simulink model ""  (R2020b)
settings: Solver=VariableStepAuto  StartTime=0.0  StopTime=10  FixedStep=0.00001  MaxStep=1e-3  RelTol=1e-3
undefined symbols (not defined in the file): h
settings Model: Creator=jofr  LastModifiedBy=jofr
settings DataIOCC: LimitDataPoints=on  SaveFormat=Array  SignalLoggingSaveFormat=ModelDataLogs  ReturnWorkspaceOutputs=off
settings OptimizationCC: BlockReduction=off  BooleanDataType=off  LifeSpan=inf
settings DebuggingCC: SaveWithParameterizedLinksMsg=none  UnderspecifiedInitializationDetection=Classic  MergeDetectMultiDrivingBlocksExec=none  SignalResolutionControl=TryResolveAllWithWarning  MultiTaskDSMMsg=warning  MultiTaskCondExecSysMsg=none  SFUnexpectedBacktrackingDiag=warning  SFNoUnconditionalDefaultTransitionDiag=warning  SFExecutionAtInitializationDiag=none  ArithmeticOperatorsInVariantConditions=warning
settings HardwareCC: ProdBitPerPointer=32  ProdBitPerSizeT=32  ProdBitPerPtrDiffT=32  ProdLargestAtomicFloat=None  ProdIntDivRoundTo=Undefined  ProdEndianess=Unspecified  ProdWordSize=32  ProdHWDeviceType=32-bit Generic  TargetUnknown=on
settings ModelReferenceCC: PropagateSignalLabelsOutOfModel=off
settings SFSimCC: SimUseLocalCustomCode=off  CustomCodeUndefinedFunction=UseInterfaceOnly
settings RTWCC: RTWUseLocalCustomCode=off
settings CodeAppCC: StateflowObjectComments=on
settings GRTTargetCC: TargetLangStandard=C89/C90 (ANSI)
settings ConfigComp: CovMetricSettings=dw  CovSaveCumulativeToWorkspaceVar=on  CovSaveSingleToWorkspaceVar=on  CovExternalEMLEnable=off

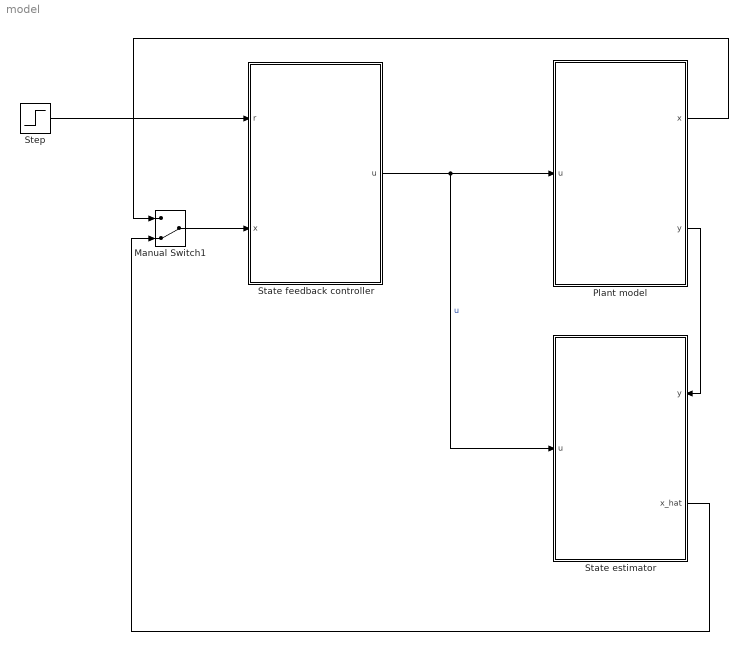
== system model ==
  Manual Switch1 : ManualSwitch  CurrentSetting=0
  Plant model : Subsystem
  State estimator : Subsystem
      settings: PortSchema="{\"entries\":[{\"content\":{\"sides\":[{\"content\":{\"connectorIds\":[\"In1\"]},\"type\":\"ConnectorPlacement.EquallySpacedRectSide\",\"uuid\":\"c417f3d4-912d-40bf-9a3a-53ea69fe223c\"},{\"content\":{\"connectorIds\":[\"In2\",\"Out1\"],\"side\":\"RIGHT\"},\"type\":\"ConnectorPlacement.EquallySpacedRectSide\",\"uuid\":\"4e25e672-d4ae-48e6-baf9-37985f0fdcbd\"},{\"content\":{\"connectorIds\":[],\"side\":\"TOP\"},\"type\":\"ConnectorPlacement.EquallySpacedRectSide\",\"uuid\":\"19dfc206-a33d-4b15-9300-bad270a3e9d6\"},{\"content\":{\"connectorIds\":[],\"side\":\"HIDDEN\"},\"type\":\"ConnectorPlacement.EquallySpacedRectSide\",\"uuid\":\"ab455fac-7bff-4c9f-9be5-2f044e5e011f\"}]},\"type\":\"ConnectorPlacement.EquallySpacedConnector\",\"uuid\":\"aea33454-8eab-4b9c-b4de-a2355e2c58aa\"}],\"packageUris\":[\"http://schema.mathworks.com/mf0/Connector/R2020b\"],\"version\":\"1.0\"}"
  State feedback controller : Subsystem
  Step : Step  Time=5  SampleTime=0
  wires:
  Plant model/1(x) -> Manual Switch1/1
  Step/1 -> State feedback controller/1(r)
  State feedback controller/1(u) -> State estimator/1(u), Plant model/1(u)  "u"
  Plant model/2(y) -> State estimator/2(y)
  Manual Switch1/1 -> State feedback controller/2(x)
  State estimator/1(x_hat) -> Manual Switch1/2

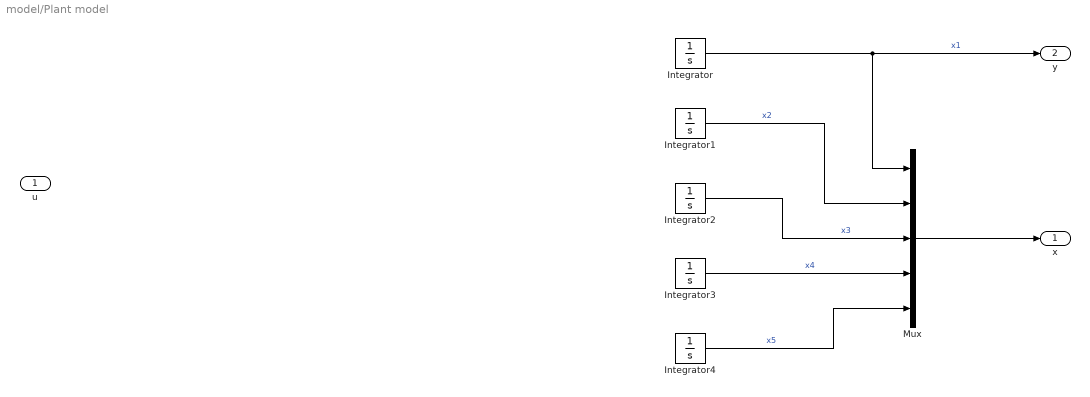
== system model/Plant model ==
  u : Inport
  Integrator{,1..4} (5 alike) : Integrator
  Mux : Mux  Inputs=5
  x : Outport
  y : Outport  Port=2
  wires:
  Integrator3/1 -> Mux/4  "x4"
  Integrator2/1 -> Mux/3  "x3"
  Integrator/1 -> Mux/1, y/1  "x1"
  Mux/1 -> x/1
  Integrator1/1 -> Mux/2  "x2"
  Integrator4/1 -> Mux/5  "x5"

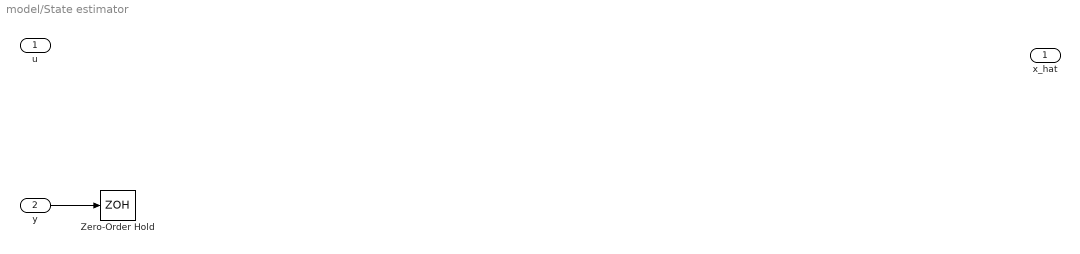
== system model/State estimator ==
  u : Inport
  y : Inport  Port=2
  Zero-Order Hold : ZeroOrderHold  SampleTime=h
  x_hat : Outport
  wires:
  y/1 -> Zero-Order Hold/1

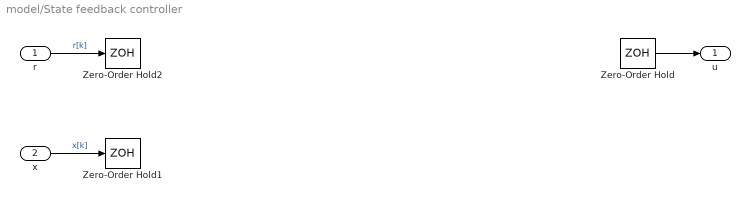
== system model/State feedback controller ==
  r : Inport
  x : Inport  Port=2
  Zero-Order Hold : ZeroOrderHold  SampleTime=h
  Zero-Order Hold1 : ZeroOrderHold  SampleTime=h
  Zero-Order Hold2 : ZeroOrderHold  SampleTime=h
  u : Outport
  wires:
  x/1 -> Zero-Order Hold1/1  "x[k]"
  r/1 -> Zero-Order Hold2/1  "r[k]"
  Zero-Order Hold/1 -> u/1
